simulink subsystem "AS_SensorBank"  (R2022a)
settings: Solver=VariableStepAuto  StartTime=0.0  StopTime=10.0  RelTol=1e-3
undefined symbols (not defined in the file): Blower_OutputDia, cmH2O_to_Pa, O2_OutputDia, O2Atmosfpere, PIDiameter
libraries: fl_lib x10, nesl_utility x7, SimscapeFluids_lib x1
settings Model: Creator=CSN-Simulation  LastModifiedBy=smith
settings DebuggingCC: UnconnectedInputMsg=warning  UnconnectedOutputMsg=warning  UnconnectedLineMsg=warning
settings RTWCC: DLArmComputeVersion=19.05

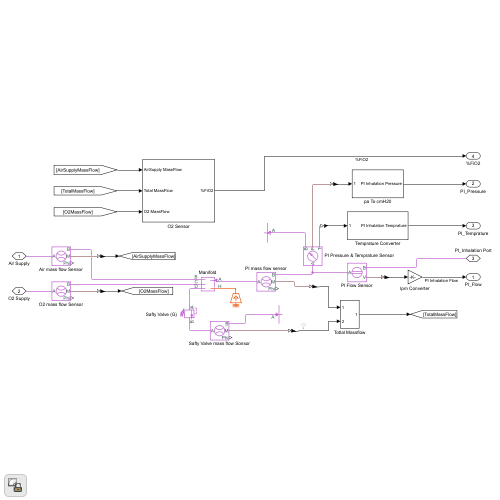
[thumbnail: Simulink's stored preview of the top-level diagram]
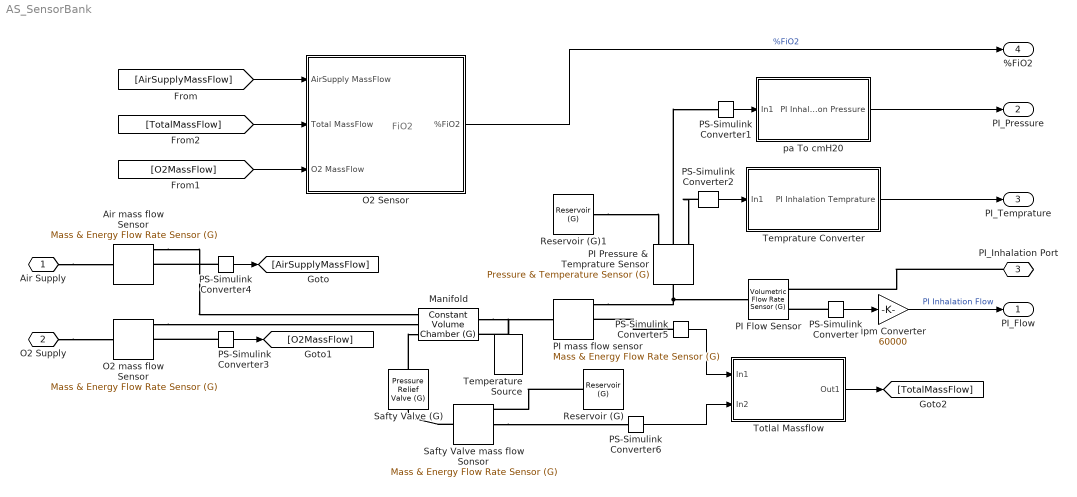
== system AS_SensorBank ==
  note: FiO2
  Air mass flow Sensor : fl_lib/Gas/Sensors/Mass & Energy Flow Rate Sensor (G)
      settings: SourceProductBaseCode=SS  InternalSimscapePortConfiguration="{\"Bottom\":[],\"Left\":[{\"id\":\"A\",\"label\":\"A\",\"type\":\"foundation.gas.gas\"}],\"Right\":[{\"id\":\"B\",\"label\":\"B\",\"type\":\"foundation.gas.gas\"},{\"id\":\"M\",\"label\":\"M\",\"type\":\"output\"},{\"id\":\"PHI\",\"label\":\"Phi\",\"type\":\"output\"}],\"Top\":[]}"
  Manifold : fl_lib/Gas/Elements/Constant Volume Chamber (G)  volume=V_SensorBank mm^3  num_ports=foundation.enum.num_ports.four  area_A=pi*(PIDiameter/2)^2 mm^2  area_B=pi*(Blower_OutputDia/2)^2 mm^2  area_C=pi*(O2_OutputDia/2)^2 mm^2  area_D=pi*(PIDiameter/2)^2 mm^2  p_I_specify=off  p_I_priority=High  p_I=P_max Pa  p_I_nominal_specify=off  p_I_nominal_unit=MPa  p_I_nominal_value=1  T_I_specify=off  T_I_priority=High  T_I=T_room degC  T_I_nominal_specify=off  T_I_nominal_unit=K  T_I_nominal_value=1  rho_chamber_specify=off  rho_chamber_priority=None  rho_chamber=1.2 kg/m^3  rho_chamber_nominal_specify=off  rho_chamber_nominal_unit=kg/m^3  rho_chamber_nominal_value=1
      settings: SourceProductBaseCode=SS  InternalSimscapePortConfiguration="{\"Bottom\":[],\"Left\":[{\"id\":\"A\",\"label\":\"A\",\"type\":\"foundation.gas.gas\"},{\"id\":\"H\",\"label\":\"H\",\"type\":\"foundation.thermal.thermal\"}],\"Right\":[{\"id\":\"B\",\"label\":\"B\",\"type\":\"foundation.gas.gas\"},{\"id\":\"C\",\"label\":\"C\",\"type\":\"foundation.gas.gas\"},{\"id\":\"D\",\"label\":\"D\",\"type\":\"foundation.gas.gas\"}],\"Top\":[]}"
  O2 Sensor : Subsystem
  O2 mass flow Sensor : fl_lib/Gas/Sensors/Mass & Energy Flow Rate Sensor (G)
      settings: SourceProductBaseCode=SS  InternalSimscapePortConfiguration="{\"Bottom\":[],\"Left\":[{\"id\":\"A\",\"label\":\"A\",\"type\":\"foundation.gas.gas\"}],\"Right\":[{\"id\":\"B\",\"label\":\"B\",\"type\":\"foundation.gas.gas\"},{\"id\":\"M\",\"label\":\"M\",\"type\":\"output\"},{\"id\":\"PHI\",\"label\":\"Phi\",\"type\":\"output\"}],\"Top\":[]}"
  PI Flow Sensor : fl_lib/Gas/Sensors/Volumetric Flow Rate Sensor (G)
      settings: SourceProductBaseCode=SS  InternalSimscapePortConfiguration="{\"Bottom\":[],\"Left\":[{\"id\":\"A\",\"label\":\"A\",\"type\":\"foundation.gas.gas\"}],\"Right\":[{\"id\":\"B\",\"label\":\"B\",\"type\":\"foundation.gas.gas\"},{\"id\":\"V\",\"label\":\"V\",\"type\":\"output\"}],\"Top\":[]}"
  PI Pressure & Temprature Sensor : fl_lib/Gas/Sensors/Pressure & Temperature Sensor (G)
      settings: SourceProductBaseCode=SS  InternalSimscapePortConfiguration="{\"Bottom\":[],\"Left\":[{\"id\":\"A\",\"label\":\"A\",\"type\":\"foundation.gas.gas\"}],\"Right\":[{\"id\":\"B\",\"label\":\"B\",\"type\":\"foundation.gas.gas\"},{\"id\":\"P\",\"label\":\"P\",\"type\":\"output\"},{\"id\":\"T\",\"label\":\"T\",\"type\":\"output\"}],\"Top\":[]}"
  PI mass flow sensor : fl_lib/Gas/Sensors/Mass & Energy Flow Rate Sensor (G)
      settings: SourceProductBaseCode=SS  InternalSimscapePortConfiguration="{\"Bottom\":[],\"Left\":[{\"id\":\"A\",\"label\":\"A\",\"type\":\"foundation.gas.gas\"}],\"Right\":[{\"id\":\"B\",\"label\":\"B\",\"type\":\"foundation.gas.gas\"},{\"id\":\"M\",\"label\":\"M\",\"type\":\"output\"},{\"id\":\"PHI\",\"label\":\"Phi\",\"type\":\"output\"}],\"Top\":[]}"
  PS-Simulink Converter{,1..6} (7 alike) : nesl_utility/PS-Simulink Converter  PhysicalDomain=network_engine_domain  SubClassName=ps_output  LeftPortType=input  RightPortType=output  PseudoPeriodic=off  Frequencies=[]  VectorFormat=1-D array  Unit=inherit  AffineConversion=off
      settings: SourceProductBaseCode=PW,SS
  Reservoir (G) : fl_lib/Gas/Elements/Reservoir (G)  pressure_spec=foundation.enum.pressure_spec.atmospheric  reservoir_pressure=0.101325 MPa  reservoir_temperature=293.15 K  area_A=pi*(O2_OutputDia/2)^2 mm^2
      settings: SourceProductBaseCode=SS
  Reservoir (G)1 : fl_lib/Gas/Elements/Reservoir (G)  pressure_spec=foundation.enum.pressure_spec.atmospheric  reservoir_pressure=0.101325 MPa  reservoir_temperature=293.15 K  area_A=0.01 m^2
      settings: SourceProductBaseCode=SS
  Safty Valve (G) : SimscapeFluids_lib/Gas/Valves & Orifices/Pressure Control Valves/Pressure Relief Valve (G)  pressure_spec=fluids.gas.enum.pressure_control_spec.pA  p_set_gauge=P_max_Gauge Pa  p_set_differential=0 MPa  p_range=0.1 Pa  iso_cond_spec=fluids.gas.enum.iso_cond_spec.area  iso_opening_spec=fluids.gas.enum.iso_opening_spec.linear  C_max=1.6 l/s/bar  C_min=1e-5 l/s/bar  B_crit=0.3  p_control_C_TLU=[0.2 : 0.2 : 1.2] MPa  C_TLU=[1e-05, .32, .64, .96, 1.28, 1.6] l/s/bar  B_crit_TLU=0.3 * ones(1, 6)  m=0.5  Cv_max=0.4  Cv_min=1e-6  p_control_Cv_TLU=[0.2 : 0.2 : 1.2] MPa  Cv_TLU=[1e-06, .08, .16, .24, .32, .4]  Kv_max=0.3  Kv_min=1e-6  p_control_Kv_TLU=[0.2 : 0.2 : 1.2] MPa  Kv_TLU=[1e-06, .06, .12, .18, .24, .3]  area_max=pi*((PIDiameter-1)/2)^2 mm^2  area_leak=1e-12 mm^2  p_control_area_TLU=[0.2 : 0.2 : 1.2] MPa  restriction_area_TLU=[1e-10, 2e-06, 4e-06, 6e-06, 8e-06, 1e-05] m^2  area=pi*(PIDiameter/2)^2 mm^2  smoothing_factor=0  B_lam=0.999  T0=T_room degC  rho0=1.185 kg/m^3
      settings: SourceProductBaseCode=SH  InternalSimscapePortConfiguration="{\"Bottom\":[],\"Left\":[{\"id\":\"A\",\"label\":\"A\",\"type\":\"foundation.gas.gas\"}],\"Right\":[{\"id\":\"B\",\"label\":\"B\",\"type\":\"foundation.gas.gas\"}],\"Top\":[]}"
  Safty Valve mass flow Sonsor : fl_lib/Gas/Sensors/Mass & Energy Flow Rate Sensor (G)
      settings: SourceProductBaseCode=SS  InternalSimscapePortConfiguration="{\"Bottom\":[],\"Left\":[{\"id\":\"A\",\"label\":\"A\",\"type\":\"foundation.gas.gas\"}],\"Right\":[{\"id\":\"B\",\"label\":\"B\",\"type\":\"foundation.gas.gas\"},{\"id\":\"M\",\"label\":\"M\",\"type\":\"output\"},{\"id\":\"PHI\",\"label\":\"Phi\",\"type\":\"output\"}],\"Top\":[]}"
  Temperature Source : fl_lib/Thermal/Thermal Sources/Temperature Source  temperature=T_room degC
  Temprature Converter : Subsystem
  Totlal Massflow : Subsystem
  lpm Converter : Gain  Gain=60000
  pa To cmH20 : Subsystem
  Air Supply : PMIOPort  Side=Left
  O2 Supply : PMIOPort  Port=2  Side=Left
  PI_Inhalation Port : PMIOPort  Port=3  Side=Right
  PI_Flow : Outport
  PI_Pressure : Outport  Port=2
  PI_Temprature : Outport  Port=3
  %FiO2 : Outport  Port=4
  wires:
  pa To cmH20/1(PI Inhalation Pressure) -> PI_Pressure/1
  PS-Simulink Converter1/1 -> pa To cmH20/1(In1)
  Totlal Massflow/1(Out1) -> [TotalMassFlow]
  PS-Simulink Converter6/1 -> Totlal Massflow/2(In2)
  PS-Simulink Converter5/1 -> Totlal Massflow/1(In1)
  PS-Simulink Converter/1 -> lpm Converter/1
  lpm Converter/1 -> PI_Flow/1  "PI Inhalation Flow"
  O2 Sensor/1(%FiO2) -> %FiO2/1  "%FiO2"
  PS-Simulink Converter4/1 -> [AirSupplyMassFlow]
  [AirSupplyMassFlow] -> O2 Sensor/1(AirSupply MassFlow)
  PS-Simulink Converter3/1 -> [O2MassFlow]
  [O2MassFlow] -> O2 Sensor/3(O2 MassFlow)
  [TotalMassFlow] -> O2 Sensor/2(Total MassFlow)
  PS-Simulink Converter2/1 -> Temprature Converter/1(In1)
  Temprature Converter/1(PI Inhalation Temprature) -> PI_Temprature/1
  connections:
  PI Pressure & Temprature Sensor/LConn1 -- PI Flow Sensor/LConn1 -- PI mass flow sensor/RConn1
  Safty Valve mass flow Sonsor/RConn2 -- PS-Simulink Converter6/LConn1
  Safty Valve mass flow Sonsor/LConn1 -- Safty Valve (G)/RConn1
  Safty Valve (G)/LConn1 -- Manifold/RConn3
  Air mass flow Sensor/RConn1 -- Manifold/RConn1
  PS-Simulink Converter5/LConn1 -- PI mass flow sensor/RConn2
  Manifold/LConn1 -- PI mass flow sensor/LConn1
  PS-Simulink Converter4/LConn1 -- Air mass flow Sensor/RConn2
  PS-Simulink Converter3/LConn1 -- O2 mass flow Sensor/RConn2
  O2 mass flow Sensor/RConn1 -- Manifold/RConn2
  Air Supply/RConn1 -- Air mass flow Sensor/LConn1
  O2 Supply/RConn1 -- O2 mass flow Sensor/LConn1
  PS-Simulink Converter2/LConn1 -- PI Pressure & Temprature Sensor/RConn3
  PI Pressure & Temprature Sensor/RConn2 -- PS-Simulink Converter1/LConn1
  PI_Inhalation Port/RConn1 -- PI Flow Sensor/RConn1
  PS-Simulink Converter/LConn1 -- PI Flow Sensor/RConn2
  Temperature Source/LConn1 -- Manifold/LConn2
  Reservoir (G)/LConn1 -- Safty Valve mass flow Sonsor/RConn1
  Reservoir (G)1/LConn1 -- PI Pressure & Temprature Sensor/RConn1

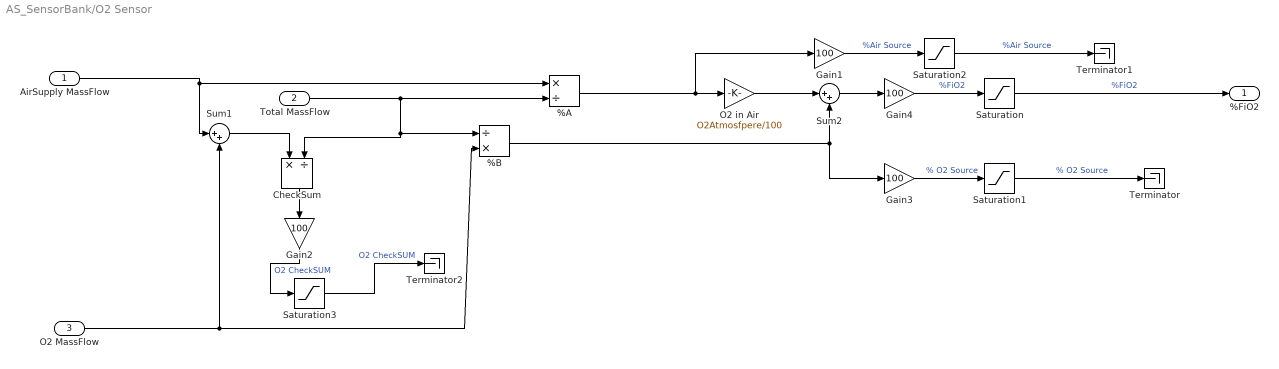
== system AS_SensorBank/O2 Sensor ==
  AirSupply MassFlow : Inport
  Total MassFlow : Inport  Port=2
  O2 MassFlow : Inport  Port=3
  %A : Product  Inputs=*/
  %B : Product  Inputs=/*
  CheckSum : Product  Inputs=*/
  Gain{1..4} (4 alike) : Gain  Gain=100
  O2 in Air : Gain  Gain=O2Atmosfpere/100
  Saturation : Saturate  UpperLimit=100  LowerLimit=0
  Saturation1 : Saturate  UpperLimit=100  LowerLimit=0
  Saturation2 : Saturate
  Saturation3 : Saturate  UpperLimit=100  LowerLimit=-100
  Sum1 : Sum  Inputs=|++
  Sum2 : Sum  Inputs=|++
  Terminator : Terminator
  Terminator1 : Terminator
  Terminator2 : Terminator
  %FiO2 : Outport
  wires:
  O2 MassFlow/1 -> %B/2, Sum1/2
  Total MassFlow/1 -> %B/1, CheckSum/2, %A/2
  Saturation1/1 -> Terminator/1  "% O2 Source"
  Sum2/1 -> Gain4/1
  Saturation3/1 -> Terminator2/1  "O2 CheckSUM"
  Sum1/1 -> CheckSum/1
  Saturation2/1 -> Terminator1/1  "%Air Source"
  CheckSum/1 -> Gain2/1
  %A/1 -> O2 in Air/1, Gain1/1
  AirSupply MassFlow/1 -> %A/1, Sum1/1
  Saturation/1 -> %FiO2/1  "%FiO2"
  %B/1 -> Sum2/2, Gain3/1
  O2 in Air/1 -> Sum2/1
  Gain4/1 -> Saturation/1  "%FiO2"
  Gain3/1 -> Saturation1/1  "% O2 Source"
  Gain1/1 -> Saturation2/1  "%Air Source"
  Gain2/1 -> Saturation3/1  "O2 CheckSUM"

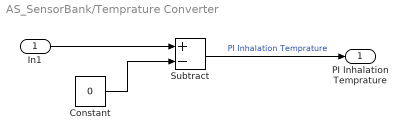
== system AS_SensorBank/Temprature Converter ==
  In1 : Inport
  Constant : Constant  Value=0
  Subtract : Sum  Inputs=+-
  PI Inhalation Temprature : Outport
  wires:
  In1/1 -> Subtract/1
  Subtract/1 -> PI Inhalation Temprature/1  "PI Inhalation Temprature"
  Constant/1 -> Subtract/2

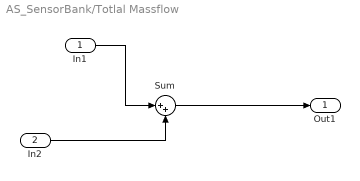
== system AS_SensorBank/Totlal Massflow ==
  In1 : Inport
  In2 : Inport  Port=2
  Sum : Sum  Inputs=|++
  Out1 : Outport
  wires:
  In1/1 -> Sum/1
  Sum/1 -> Out1/1
  In2/1 -> Sum/2

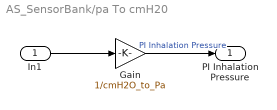
== system AS_SensorBank/pa To cmH20 ==
  In1 : Inport
  Gain : Gain  Gain=1/cmH2O_to_Pa
  PI Inhalation Pressure : Outport
  wires:
  Gain/1 -> PI Inhalation Pressure/1  "PI Inhalation Pressure"
  In1/1 -> Gain/1
